simulink model "pushpull_lc_fig"  (R2023b)
settings: Solver=VariableStepAuto  StartTime=0.0  StopTime=10.0  RelTol=1e-3
libraries: spsSeriesRLCBranchLib x10, spsGroundLib x4, spsMosfetLib x2, spsControlledVoltageSourceLib x1, spsCurrentMeasurementLib x1, spsMultiWindingTransformerLib x1, spsPowerLib x1, spsVariableResistorLib x1, spsVoltageMeasurementLib x1
settings Model: Creator=ASUS  LastModifiedBy=ASUS

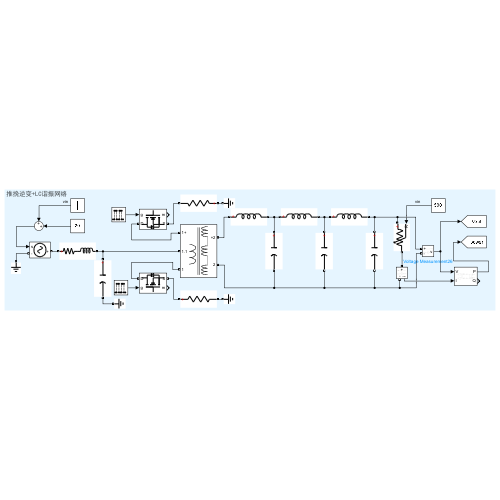
[thumbnail: Simulink's stored preview of the top-level diagram]
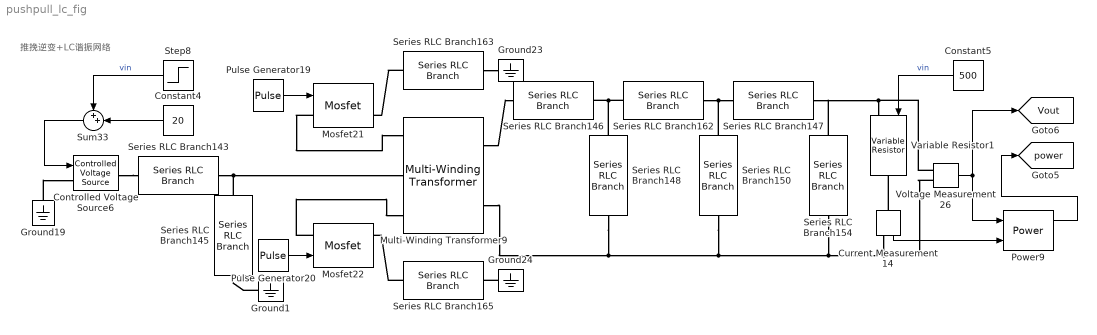
== system pushpull_lc_fig ==
  note: 推挽逆变+LC谐振网络
  Constant4 : Constant  Value=20  SampleTime=1e-8
  Constant5 : Constant  Value=500
  Controlled Voltage Source6 : spsControlledVoltageSourceLib/Controlled Voltage Source  Initialize=off  Source_Type=DC  Amplitude=20  Phase=0  Frequency=0  Measurements=None
  Current Measurement14 : spsCurrentMeasurementLib/Current Measurement  PhasorSimulation=off  OutputType=Complex  PSBequivalent=0
  Ground{1,19,23..24} (4 alike) : spsGroundLib/Ground  LConnTagsString=a
  Mosfet21 : spsMosfetLib/Mosfet  Ron=0.1  Lon=0  Rd=0.01  Vfd=0  IC=0  Rs=1e5  Cs=inf  Measurements=on
  Mosfet22 : spsMosfetLib/Mosfet  Ron=0.1  Lon=0  Rd=0.01  Vfd=0  IC=0  Rs=1e5  Cs=inf  Measurements=on
  Multi-Winding Transformer9 : spsMultiWindingTransformerLib/Multi-Winding Transformer  LeftWindings=1  RightWindings=1  TappedWindings=taps on upper left winding  NumberOfTaps=1  SetSaturation=off  Hysteresis=off  DataFile='hysteresis.mat'  Measurements=None  UNITS=SI  NominalPower=[120 400000]  NominalVoltages=[2 4]  WindingResistances=[0 0]  WindingInductances=[0 0]  Rm=inf  Lm=inf  Saturation=[0 0;2.8284e-05 0.0097234;0.011785 0.012316]  SpecifyInitialFlux=off  InitialFlux=0  BreakLoop=off  DiscreteSolver=Trapezoidal iterative  DataType=on  TransfoNumber=1
      settings: LibrarySourceBlock=|
      | sps_lib/Power Grid Elements/Multi-Winding
      | Transformer
  Power9 : spsPowerLib/Power  Freq=350000  Vinit=[1, 0]  Iinit=[1, 0]  Ts=1e-8
  Pulse Generator19 : DiscretePulseGenerator  Amplitude=12  Period=286  PulseWidth=133  SampleTime=1e-8
  Pulse Generator20 : DiscretePulseGenerator  Amplitude=12  Period=286  PulseWidth=133  PhaseDelay=143  SampleTime=1e-8
  Series RLC Branch143 : spsSeriesRLCBranchLib/Series RLC Branch  LConnTagsString=__new0  RConnTagsString=__new0  BranchType=RL  Resistance=2  Inductance=2.2e-6  SetiL0=off  InitialCurrent=0  Capacitance=1e-6  Setx0=off  InitialVoltage=0  Measurements=None
  Series RLC Branch145 : spsSeriesRLCBranchLib/Series RLC Branch  LConnTagsString=__new0  RConnTagsString=__new0  BranchType=C  Resistance=1  Inductance=220e-6  SetiL0=off  InitialCurrent=0  Capacitance=10e-6  Setx0=off  InitialVoltage=0  Measurements=None
  Series RLC Branch146 : spsSeriesRLCBranchLib/Series RLC Branch  LConnTagsString=__new0  RConnTagsString=__new0  BranchType=L  Resistance=1  Inductance=150e-6  SetiL0=off  InitialCurrent=0  Capacitance=1e-6  Setx0=off  InitialVoltage=0  Measurements=None
  Series RLC Branch147 : spsSeriesRLCBranchLib/Series RLC Branch  LConnTagsString=__new0  RConnTagsString=__new0  BranchType=L  Resistance=1  Inductance=150e-6  SetiL0=off  InitialCurrent=0  Capacitance=1e-6  Setx0=off  InitialVoltage=0  Measurements=None
  Series RLC Branch148 : spsSeriesRLCBranchLib/Series RLC Branch  LConnTagsString=__new0  RConnTagsString=__new0  BranchType=C  Resistance=1  Inductance=220e-6  SetiL0=off  InitialCurrent=0  Capacitance=1.451e-9  Setx0=off  InitialVoltage=0  Measurements=None
  Series RLC Branch150 : spsSeriesRLCBranchLib/Series RLC Branch  LConnTagsString=__new0  RConnTagsString=__new0  BranchType=C  Resistance=1  Inductance=220e-6  SetiL0=off  InitialCurrent=0  Capacitance=180e-12  Setx0=off  InitialVoltage=0  Measurements=None
  Series RLC Branch154 : spsSeriesRLCBranchLib/Series RLC Branch  LConnTagsString=__new0  RConnTagsString=__new0  BranchType=C  Resistance=1  Inductance=220e-6  SetiL0=off  InitialCurrent=0  Capacitance=51e-12  Setx0=off  InitialVoltage=0  Measurements=None
  Series RLC Branch162 : spsSeriesRLCBranchLib/Series RLC Branch  LConnTagsString=__new0  RConnTagsString=__new0  BranchType=L  Resistance=1  Inductance=220e-6  SetiL0=off  InitialCurrent=0  Capacitance=1e-6  Setx0=off  InitialVoltage=0  Measurements=None
  Series RLC Branch163 : spsSeriesRLCBranchLib/Series RLC Branch  LConnTagsString=__new0  RConnTagsString=__new0  BranchType=R  Resistance=0.02  Inductance=220e-6  SetiL0=off  InitialCurrent=0  Capacitance=180e-12  Setx0=off  InitialVoltage=0  Measurements=None
  Series RLC Branch165 : spsSeriesRLCBranchLib/Series RLC Branch  LConnTagsString=__new0  RConnTagsString=__new0  BranchType=R  Resistance=0.02  Inductance=220e-6  SetiL0=off  InitialCurrent=0  Capacitance=180e-12  Setx0=off  InitialVoltage=0  Measurements=None
  Step8 : Step  Time=0.0005  After=20  SampleTime=1e-8
  Sum33 : Sum  Inputs=++|
  Variable Resistor1 : spsVariableResistorLib/Variable Resistor  Rabsmin=0
      settings: LibrarySourceBlock=sps_lib/Passives/Variable Resistor
  Voltage Measurement26 : spsVoltageMeasurementLib/Voltage Measurement  PhasorSimulation=off  OutputType=Complex  PSBequivalent=0
  tag scope: Vout=global, power=global
  wires:
  Voltage Measurement26/1 -> Power9/1, [Vout]
  Current Measurement14/1 -> Power9/2
  Pulse Generator20/1 -> Mosfet22/1
  Power9/1 -> [power]
  Constant5/1 -> Variable Resistor1/1  "vin"
  Pulse Generator19/1 -> Mosfet21/1
  Step8/1 -> Sum33/1  "vin"
  Sum33/1 -> Controlled Voltage Source6/1
  Constant4/1 -> Sum33/2
  connections:
  Voltage Measurement26/LConn1 -- Series RLC Branch154/LConn1 -- Series RLC Branch147/RConn1 -- Variable Resistor1/LConn1
  Series RLC Branch148/RConn1 -- Multi-Winding Transformer9/RConn2 -- Series RLC Branch150/RConn1 -- Series RLC Branch154/RConn1 -- Voltage Measurement26/LConn2 -- Current Measurement14/RConn1
  Series RLC Branch162/RConn1 -- Series RLC Branch150/LConn1 -- Series RLC Branch147/LConn1
  Series RLC Branch148/LConn1 -- Series RLC Branch162/LConn1 -- Series RLC Branch146/RConn1
  Mosfet22/LConn1 -- Multi-Winding Transformer9/LConn3
  Series RLC Branch165/LConn1 -- Mosfet22/RConn1
  Mosfet21/LConn1 -- Multi-Winding Transformer9/LConn1
  Current Measurement14/LConn1 -- Variable Resistor1/RConn1
  Ground24/LConn1 -- Series RLC Branch165/RConn1
  Series RLC Branch163/RConn1 -- Mosfet21/RConn1
  Series RLC Branch163/LConn1 -- Ground23/LConn1
  Multi-Winding Transformer9/RConn1 -- Series RLC Branch146/LConn1
  Controlled Voltage Source6/RConn1 -- Series RLC Branch143/LConn1
  Ground19/LConn1 -- Controlled Voltage Source6/LConn1
  Series RLC Branch143/RConn1 -- Series RLC Branch145/LConn1 -- Multi-Winding Transformer9/LConn2
  Ground1/LConn1 -- Series RLC Branch145/RConn1
